simulink model "Controlador_TCC"  (R2023b)
settings: Solver=VariableStepAuto  StartTime=0.0  StopTime=83.0  RelTol=1e-3
settings Model: Creator=Eitão  LastModifiedBy=Eitão

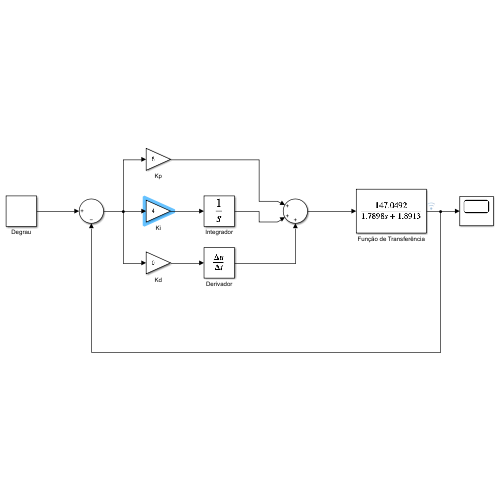
[thumbnail: Simulink's stored preview of the top-level diagram]
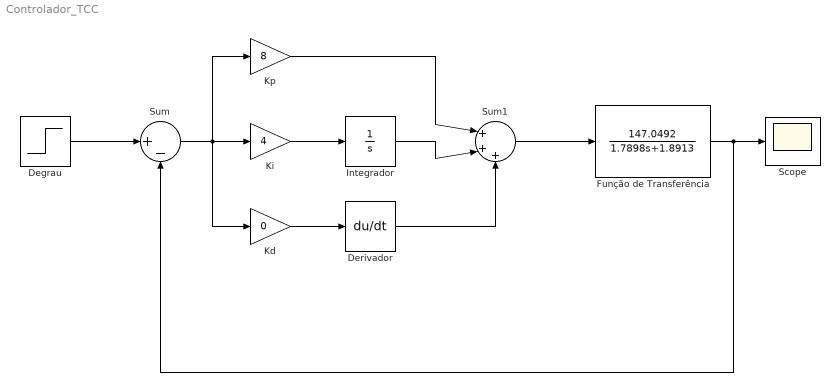
== system Controlador_TCC ==
  Degrau : Step  After=60  SampleTime=0
  Derivador : Derivative
  Função de Transferência : TransferFcn  Numerator=[147.0492]  Denominator=[1.7898 1.8913]
  Integrador : Integrator
  Kd : Gain  Gain=0
  Ki : Gain  Gain=4
  Kp : Gain  Gain=8
  Scope : Scope
  Sum : Sum  Inputs=|+-
  Sum1 : Sum  Inputs=|+++
  wires:
  Degrau/1 -> Sum/1
  Função de Transferência/1 -> Sum/2, Scope/1
  Sum/1 -> Kd/1, Kp/1, Ki/1
  Ki/1 -> Integrador/1
  Kd/1 -> Derivador/1
  Sum1/1 -> Função de Transferência/1
  Kp/1 -> Sum1/1
  Integrador/1 -> Sum1/2
  Derivador/1 -> Sum1/3
